simulink model "Simulacion_dinamica_en_DT_export"  (R2023b)
settings: Solver=VariableStepAuto  StartTime=0.0  StopTime=2.5  MaxStep=6e-5  RelTol=1e-3
undefined symbols (not defined in the file): alpha_cu, b_eq, C_ts, id0, J_eq, k_l, L_d, L_ls, L_q, lambda_m, magnitude, P_p, r, R_sREF, R_ts_amb, T_amb, T_sREF
libraries: SignalEditorBlockLib x2, dspsigops x1
settings Model: Creator=tomas  LastModifiedBy=tomas

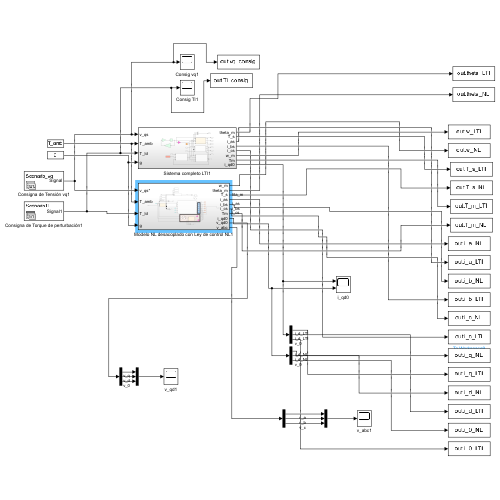
[thumbnail: Simulink's stored preview of the top-level diagram]
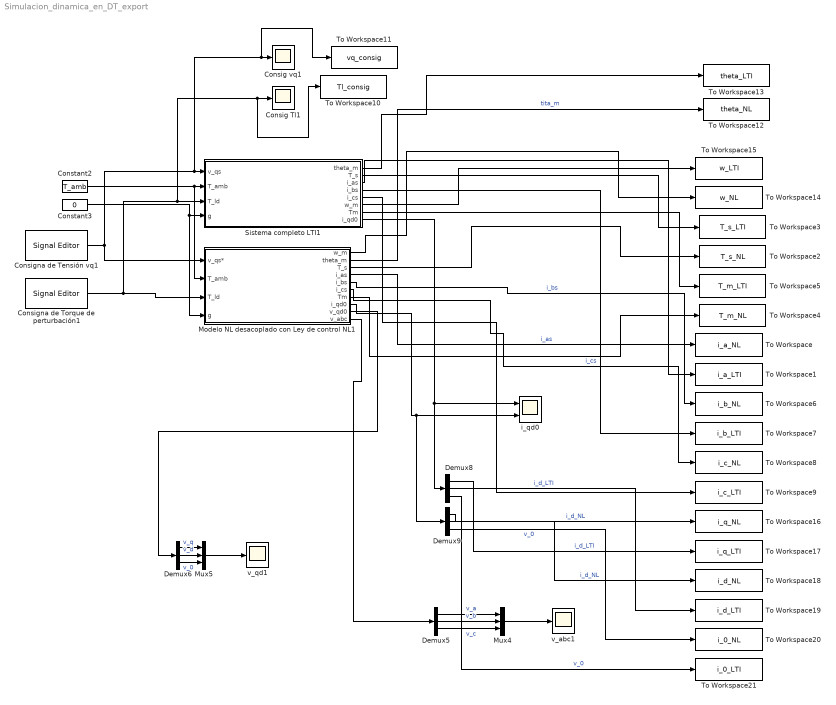
== system Simulacion_dinamica_en_DT_export ==
  Consig Tl1 : Scope
  Consig vq1 : Scope
  Consigna de Tensión vq1 : SignalEditorBlockLib/Signal Editor  FileName=D:\Facu\Final AyME\Final-AyME\Simulink_LA\Simulacion\Señales\senial_vq.mat  ActiveScenario=Scenario_vq  ActiveSignal=Signal  IsBus=off  OutputBusObjectStr=Bus: BusObject  SampleTime=0  Interpolate=off  ZeroCross=off  OutputAfterFinalValue=Setting to zero  Unit=inherit  PreserveSignalName=on  ApplySigPropsToAllScenarios=on  ApplySigPropsToAllSignals=off
  Consigna de Torque de perturbación1 : SignalEditorBlockLib/Signal Editor  FileName=D:\Facu\Final AyME\Final-AyME\Simulink_LA\Simulacion\Señales\Signal_Tl.mat  ActiveScenario=ScenarioTl  ActiveSignal=Signal1  IsBus=off  OutputBusObjectStr=Bus: BusObject  SampleTime=0  Interpolate=off  ZeroCross=off  OutputAfterFinalValue=Setting to zero  Unit=inherit  PreserveSignalName=on  ApplySigPropsToAllScenarios=on  ApplySigPropsToAllSignals=off
  Constant2 : Constant  Value=T_amb
  Constant3 : Constant  Value=0
  Demux{5..6,8..9} (4 alike) : Demux  Outputs=3
  Modelo NL desacoplado con Ley de control NL1 : Subsystem
  Mux4 : Mux  Inputs=3
  Mux5 : Mux  Inputs=3
  Sistema completo LTI1 : Subsystem
  To Workspace : ToWorkspace  VariableName=i_a_NL  SaveFormat=Structure With Time  SampleTime=-1
  To Workspace1 : ToWorkspace  VariableName=i_a_LTI  SaveFormat=Structure With Time  SampleTime=-1
  To Workspace10 : ToWorkspace  VariableName=Tl_consig  SaveFormat=Structure With Time  SampleTime=-1
  To Workspace11 : ToWorkspace  VariableName=vq_consig  SaveFormat=Structure With Time  SampleTime=-1
  To Workspace12 : ToWorkspace  VariableName=theta_NL  SaveFormat=Structure With Time  SampleTime=-1
  To Workspace13 : ToWorkspace  VariableName=theta_LTI  SaveFormat=Structure With Time  SampleTime=-1
  To Workspace14 : ToWorkspace  VariableName=w_NL  SaveFormat=Structure With Time  SampleTime=-1
  To Workspace15 : ToWorkspace  VariableName=w_LTI  SaveFormat=Structure With Time  SampleTime=-1
  To Workspace16 : ToWorkspace  VariableName=i_q_NL  SaveFormat=Structure With Time  SampleTime=-1
  To Workspace17 : ToWorkspace  VariableName=i_q_LTI  SaveFormat=Structure With Time  SampleTime=-1
  To Workspace18 : ToWorkspace  VariableName=i_d_NL  SaveFormat=Structure With Time  SampleTime=-1
  To Workspace19 : ToWorkspace  VariableName=i_d_LTI  SaveFormat=Structure With Time  SampleTime=-1
  To Workspace2 : ToWorkspace  VariableName=T_s_NL  SaveFormat=Structure With Time  SampleTime=-1
  To Workspace20 : ToWorkspace  VariableName=i_0_NL  SaveFormat=Structure With Time  SampleTime=-1
  To Workspace21 : ToWorkspace  VariableName=i_0_LTI  SaveFormat=Structure With Time  SampleTime=-1
  To Workspace3 : ToWorkspace  VariableName=T_s_LTI  SaveFormat=Structure With Time  SampleTime=-1
  To Workspace4 : ToWorkspace  VariableName=T_m_NL  SaveFormat=Structure With Time  SampleTime=-1
  To Workspace5 : ToWorkspace  VariableName=T_m_LTI  SaveFormat=Structure With Time  SampleTime=-1
  To Workspace6 : ToWorkspace  VariableName=i_b_NL  SaveFormat=Structure With Time  SampleTime=-1
  To Workspace7 : ToWorkspace  VariableName=i_b_LTI  SaveFormat=Structure With Time  SampleTime=-1
  To Workspace8 : ToWorkspace  VariableName=i_c_NL  SaveFormat=Structure With Time  SampleTime=-1
  To Workspace9 : ToWorkspace  VariableName=i_c_LTI  SaveFormat=Structure With Time  SampleTime=-1
  i_qd0 : Scope  NumInputPorts=2
  v_abc1 : Scope
  v_qd1 : Scope
  wires:
  Mux4/1 -> v_abc1/1
  Demux5/1 -> Mux4/1  "v_a"
  Sistema completo LTI1/6(w_m) -> To Workspace15/1
  Sistema completo LTI1/4(i_bs) -> To Workspace7/1
  Modelo NL desacoplado con Ley de control NL1/9(v_qd0) -> Demux6/1
  Constant2/1 -> Modelo NL desacoplado con Ley de control NL1/2(T_amb), Sistema completo LTI1/2(T_amb)
  Modelo NL desacoplado con Ley de control NL1/10(v_abc) -> Demux5/1
  Mux5/1 -> v_qd1/1
  Demux6/3 -> Mux5/3  "v_0"
  Demux6/1 -> Mux5/1  "v_q"
  Demux5/2 -> Mux4/2  "v_b"
  Modelo NL desacoplado con Ley de control NL1/7(Tm) -> To Workspace4/1
  Demux5/3 -> Mux4/3  "v_c"
  Modelo NL desacoplado con Ley de control NL1/6(i_cs) -> To Workspace8/1  "i_cs"
  Modelo NL desacoplado con Ley de control NL1/5(i_bs) -> To Workspace6/1  "i_bs"
  Sistema completo LTI1/7(Tm) -> To Workspace5/1
  Modelo NL desacoplado con Ley de control NL1/4(i_as) -> To Workspace/1  "i_as"
  Demux6/2 -> Mux5/2  "v_d"
  Modelo NL desacoplado con Ley de control NL1/1(w_m) -> To Workspace14/1
  Constant3/1 -> Modelo NL desacoplado con Ley de control NL1/4(g), Sistema completo LTI1/4(g)
  Modelo NL desacoplado con Ley de control NL1/2(theta_m) -> To Workspace12/1  "tita_m"
  Sistema completo LTI1/5(i_cs) -> To Workspace9/1
  Modelo NL desacoplado con Ley de control NL1/8(i_qd0) -> i_qd0/2, Demux9/1
  Sistema completo LTI1/8(i_qd0) -> Demux8/1, i_qd0/1
  Sistema completo LTI1/2(T_s) -> To Workspace3/1
  Modelo NL desacoplado con Ley de control NL1/3(T_s) -> To Workspace2/1
  Sistema completo LTI1/1(theta_m) -> To Workspace13/1
  Sistema completo LTI1/3(i_as) -> To Workspace1/1
  Consigna de Tensión vq1/1 -> To Workspace11/1, Consig vq1/1, Sistema completo LTI1/1(v_qs), Modelo NL desacoplado con Ley de control NL1/1(v_qs*)
  Consigna de Torque de perturbación1/1 -> Modelo NL desacoplado con Ley de control NL1/3(T_ld), To Workspace10/1, Consig Tl1/1, Sistema completo LTI1/3(T_ld)
  Demux8/1 -> To Workspace17/1  "i_d_LTI"
  Demux8/2 -> To Workspace19/1  "i_d_LTI"
  Demux8/3 -> To Workspace21/1  "v_0"
  Demux9/1 -> To Workspace16/1  "i_d_NL"
  Demux9/2 -> To Workspace18/1  "i_d_NL"
  Demux9/3 -> To Workspace20/1  "v_0"

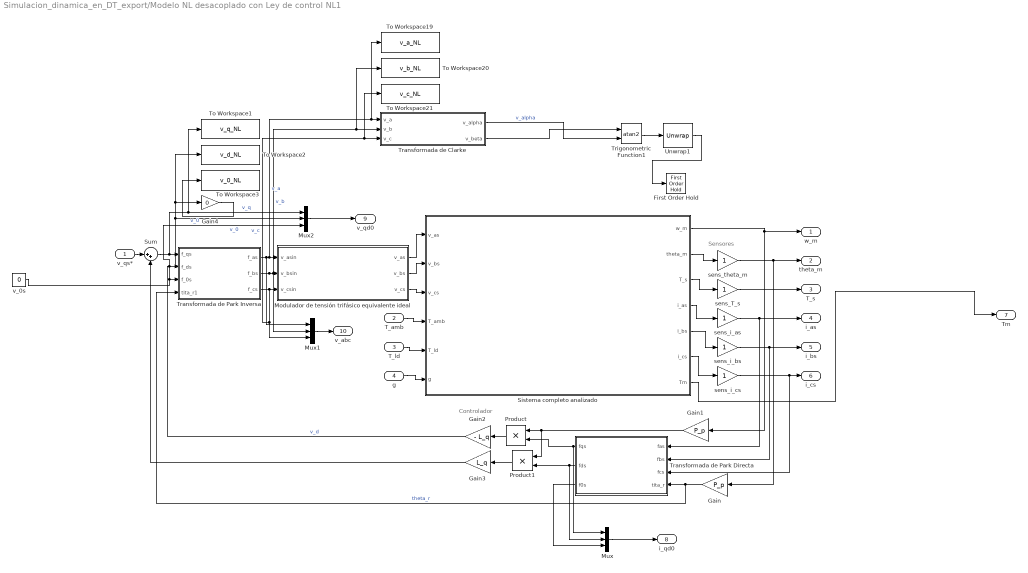
== system Simulacion_dinamica_en_DT_export/Modelo NL desacoplado con Ley de control NL1 ==
  note: Sensores
  note: Controlador
  v_qs* : Inport
  T_amb : Inport  Port=2
  T_ld : Inport  Port=3
  g : Inport  Port=4
  First Order Hold : FirstOrderHold  ErrorTolerance=inf  AllowContinuousInput=on
  Gain : Gain  Gain=P_p
  Gain1 : Gain  Gain=P_p
  Gain2 : Gain  Gain=- L_q
  Gain3 : Gain  Gain=L_q
  Gain4 : Gain  Gain=0
  Modulador de tensión trifásico equivalente ideal : MATLAB Function  TreatAsAtomicUnit=on
  Mux : Mux  Inputs=3
  Mux1 : Mux  Inputs=3
  Mux2 : Mux  Inputs=3
  Product : Product
  Product1 : Product
  "Sistema completo analizado " : Subsystem
  Sum : Sum  Inputs=|++
  To Workspace1 : ToWorkspace  VariableName=v_q_NL  SaveFormat=Structure With Time  SampleTime=-1
  To Workspace19 : ToWorkspace  VariableName=v_a_NL  SaveFormat=Structure With Time  SampleTime=-1
  To Workspace2 : ToWorkspace  VariableName=v_d_NL  SaveFormat=Structure With Time  SampleTime=-1
  To Workspace20 : ToWorkspace  VariableName=v_b_NL  SaveFormat=Structure With Time  SampleTime=-1
  To Workspace21 : ToWorkspace  VariableName=v_c_NL  SaveFormat=Structure With Time  SampleTime=-1
  To Workspace3 : ToWorkspace  VariableName=v_0_NL  SaveFormat=Structure With Time  SampleTime=-1
  Transformada de Clarke : MATLAB Function  TreatAsAtomicUnit=on
  Transformada de Park Directa : Subsystem
  Transformada de Park Inversa : Subsystem
  Trigonometric Function1 : Trigonometry  Operator=atan2
  Unwrap1 : dspsigops/Unwrap  tol=1.2*pi  InputProcessing=Columns as channels (frame based)  running=off
  sens_T_s : Gain
  sens_i_as : Gain
  sens_i_bs : Gain
  sens_i_cs : Gain
  sens_theta_m : Gain
  v_0s : Constant  Value=0
  w_m : Outport
  theta_m : Outport  Port=2
  T_s : Outport  Port=3
  i_as : Outport  Port=4
  i_bs : Outport  Port=5
  i_cs : Outport  Port=6
  Tm : Outport  Port=7
  i_qd0 : Outport  Port=8
  v_qd0 : Outport  Port=9
  v_abc : Outport  Port=10
  wires:
  "Sistema completo analizado "/5(i_bs) -> sens_i_bs/1
  Gain1/1 -> Product1/1, Product/1
  Transformada de Park Directa/3(f0s) -> Mux/3
  T_amb/1 -> "Sistema completo analizado "/4(T_amb)
  "Sistema completo analizado "/3(T_s) -> sens_T_s/1
  g/1 -> "Sistema completo analizado "/6(g)
  Modulador de tensión trifásico equivalente ideal/2(v_bs) -> "Sistema completo analizado "/2(v_bs)
  sens_T_s/1 -> T_s/1
  Transformada de Park Directa/1(fqs) -> Mux/1, Product/2
  Modulador de tensión trifásico equivalente ideal/1(v_as) -> "Sistema completo analizado "/1(v_as)
  sens_i_as/1 -> Transformada de Park Directa/1(fas), i_as/1
  "Sistema completo analizado "/6(i_cs) -> sens_i_cs/1
  "Sistema completo analizado "/4(i_as) -> sens_i_as/1
  Transformada de Park Inversa/3(f_cs) -> Mux1/3, Transformada de Clarke/3(v_c), To Workspace21/1, Modulador de tensión trifásico equivalente ideal/3(v_csin)  "v_c"
  Transformada de Park Inversa/1(f_as) -> Mux1/1, To Workspace19/1, Transformada de Clarke/1(v_a), Modulador de tensión trifásico equivalente ideal/1(v_asin)  "v_a"
  Transformada de Park Inversa/2(f_bs) -> Transformada de Clarke/2(v_b), To Workspace20/1, Mux1/2, Modulador de tensión trifásico equivalente ideal/2(v_bsin)  "v_b"
  v_qs*/1 -> Sum/1
  Product1/1 -> Gain3/1
  "Sistema completo analizado "/2(theta_m) -> sens_theta_m/1
  Transformada de Park Directa/2(fds) -> Mux/2, Product1/2
  sens_theta_m/1 -> Gain/1, theta_m/1
  sens_i_bs/1 -> Transformada de Park Directa/2(fbs), i_bs/1
  v_0s/1 -> Mux2/3, Transformada de Park Inversa/3(f_0s)  "v_0"
  Gain/1 -> Transformada de Park Inversa/4(tita_r1), Transformada de Park Directa/4(tita_r)  "theta_r"
  Gain2/1 -> To Workspace2/1, Gain4/1, Mux2/2, Transformada de Park Inversa/2(f_ds)  "v_d"
  Product/1 -> Gain2/1
  Modulador de tensión trifásico equivalente ideal/3(v_cs) -> "Sistema completo analizado "/3(v_cs)
  Sum/1 -> To Workspace1/1, Mux2/1, Transformada de Park Inversa/1(f_qs)  "v_q"
  sens_i_cs/1 -> Transformada de Park Directa/3(fcs), i_cs/1
  T_ld/1 -> "Sistema completo analizado "/5(T_ld)
  Gain3/1 -> Sum/2
  "Sistema completo analizado "/1(w_m) -> Gain1/1, w_m/1
  "Sistema completo analizado "/7(Tm) -> Tm/1
  Mux/1 -> i_qd0/1
  Mux1/1 -> v_abc/1
  Mux2/1 -> v_qd0/1
  Unwrap1/1 -> First Order Hold/1
  Transformada de Clarke/1(v_alpha) -> Trigonometric Function1/2  "v_alpha"
  Trigonometric Function1/1 -> Unwrap1/1
  Transformada de Clarke/2(v_beta) -> Trigonometric Function1/1
  Gain4/1 -> To Workspace3/1  "v_0"

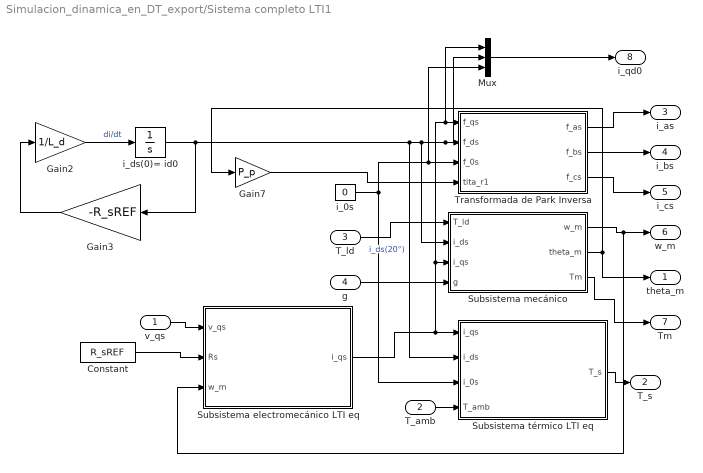
== system Simulacion_dinamica_en_DT_export/Sistema completo LTI1 ==
  v_qs : Inport
  T_amb : Inport  Port=2
  T_ld : Inport  Port=3
  g : Inport  Port=4
  Constant : Constant  Value=R_sREF
  Gain2 : Gain  Gain=1/L_d
  Gain3 : Gain  Gain=-R_sREF
  Gain7 : Gain  Gain=P_p
  Mux : Mux  Inputs=3
  Subsistema electromecánico LTI eq : Subsystem
  Subsistema mecánico : Subsystem
  Subsistema térmico LTI eq : Subsystem
  Transformada de Park Inversa : Subsystem
  i_0s : Constant  Value=0
  i_ds(0)= id0 : Integrator  InitialCondition=id0
  theta_m : Outport
  T_s : Outport  Port=2
  i_as : Outport  Port=3
  i_bs : Outport  Port=4
  i_cs : Outport  Port=5
  w_m : Outport  Port=6
  Tm : Outport  Port=7
  i_qd0 : Outport  Port=8
  wires:
  Subsistema mecánico/2(theta_m) -> theta_m/1, Gain7/1
  v_qs/1 -> Subsistema electromecánico LTI eq/1(v_qs)
  Transformada de Park Inversa/1(f_as) -> i_as/1
  T_ld/1 -> Subsistema mecánico/1(T_ld)
  Transformada de Park Inversa/2(f_bs) -> i_bs/1
  Subsistema térmico LTI eq/1(T_s) -> T_s/1
  Transformada de Park Inversa/3(f_cs) -> i_cs/1
  Subsistema mecánico/1(w_m) -> Subsistema electromecánico LTI eq/3(w_m), w_m/1
  T_amb/1 -> Subsistema térmico LTI eq/4(T_amb)
  i_0s/1 -> Subsistema térmico LTI eq/3(i_0s), Transformada de Park Inversa/3(f_0s), Mux/3
  Constant/1 -> Subsistema electromecánico LTI eq/2(Rs)
  Subsistema electromecánico LTI eq/1(i_qs) -> Subsistema mecánico/3(i_qs), Mux/1, Transformada de Park Inversa/1(f_qs), Subsistema térmico LTI eq/1(i_qs)
  Gain7/1 -> Transformada de Park Inversa/4(tita_r1)
  i_ds(0)= id0/1 -> Subsistema mecánico/2(i_ds), Mux/2, Transformada de Park Inversa/2(f_ds), Subsistema térmico LTI eq/2(i_ds), Gain3/1  "i_ds(20°)"
  Gain2/1 -> i_ds(0)= id0/1  "di/dt"
  g/1 -> Subsistema mecánico/4(g)
  Subsistema mecánico/3(Tm) -> Tm/1
  Mux/1 -> i_qd0/1
  Gain3/1 -> Gain2/1

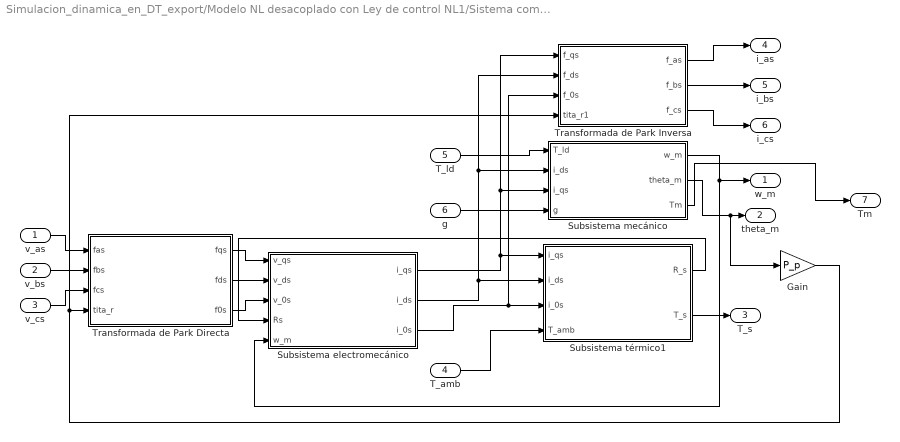
== system Simulacion_dinamica_en_DT_export/Modelo NL desacoplado con Ley de control NL1/Sistema completo analizado  ==
  v_as : Inport
  v_bs : Inport  Port=2
  v_cs : Inport  Port=3
  T_amb : Inport  Port=4
  T_ld : Inport  Port=5
  g : Inport  Port=6
  Gain : Gain  Gain=P_p
  Subsistema electromecánico : Subsystem
  Subsistema mecánico : Subsystem
  Subsistema térmico1 : Subsystem
  Transformada de Park Directa : Subsystem
  Transformada de Park Inversa : Subsystem
  w_m : Outport
  theta_m : Outport  Port=2
  T_s : Outport  Port=3
  i_as : Outport  Port=4
  i_bs : Outport  Port=5
  i_cs : Outport  Port=6
  Tm : Outport  Port=7
  wires:
  Transformada de Park Inversa/3(f_cs) -> i_cs/1
  Subsistema mecánico/1(w_m) -> w_m/1, Subsistema electromecánico/5(w_m)
  Subsistema electromecánico/3(i_0s) -> Subsistema térmico1/3(i_0s), Transformada de Park Inversa/3(f_0s)
  Transformada de Park Directa/1(fqs) -> Subsistema electromecánico/1(v_qs)
  Subsistema térmico1/2(T_s) -> T_s/1
  Transformada de Park Directa/3(f0s) -> Subsistema electromecánico/3(v_0s)
  Subsistema electromecánico/2(i_ds) -> Subsistema térmico1/2(i_ds), Transformada de Park Inversa/2(f_ds), Subsistema mecánico/2(i_ds)
  Gain/1 -> Transformada de Park Inversa/4(tita_r1), Transformada de Park Directa/4(tita_r)
  T_ld/1 -> Subsistema mecánico/1(T_ld)
  Transformada de Park Directa/2(fds) -> Subsistema electromecánico/2(v_ds)
  Transformada de Park Inversa/2(f_bs) -> i_bs/1
  v_bs/1 -> Transformada de Park Directa/2(fbs)
  T_amb/1 -> Subsistema térmico1/4(T_amb)
  Transformada de Park Inversa/1(f_as) -> i_as/1
  v_as/1 -> Transformada de Park Directa/1(fas)
  Subsistema mecánico/2(theta_m) -> Gain/1, theta_m/1
  v_cs/1 -> Transformada de Park Directa/3(fcs)
  Subsistema electromecánico/1(i_qs) -> Transformada de Park Inversa/1(f_qs), Subsistema mecánico/3(i_qs), Subsistema térmico1/1(i_qs)
  Subsistema térmico1/1(R_s) -> Subsistema electromecánico/4(Rs)
  g/1 -> Subsistema mecánico/4(g)
  Subsistema mecánico/3(Tm) -> Tm/1

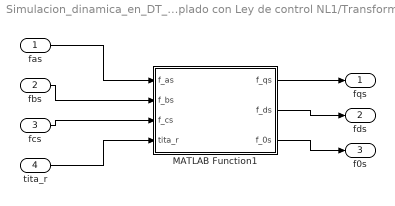
== system Simulacion_dinamica_en_DT_export/Modelo NL desacoplado con Ley de control NL1/Transformada de Park Directa ==
  fas : Inport
  fbs : Inport  Port=2
  fcs : Inport  Port=3
  tita_r : Inport  Port=4
  MATLAB Function1 : MATLAB Function  TreatAsAtomicUnit=on
  fqs : Outport
  fds : Outport  Port=2
  f0s : Outport  Port=3
  wires:
  fas/1 -> MATLAB Function1/1(f_as)
  MATLAB Function1/3(f_0s) -> f0s/1
  MATLAB Function1/2(f_ds) -> fds/1
  fbs/1 -> MATLAB Function1/2(f_bs)
  fcs/1 -> MATLAB Function1/3(f_cs)
  tita_r/1 -> MATLAB Function1/4(tita_r)
  MATLAB Function1/1(f_qs) -> fqs/1

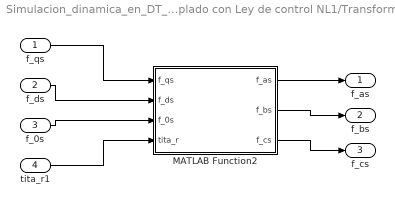
== system Simulacion_dinamica_en_DT_export/Modelo NL desacoplado con Ley de control NL1/Transformada de Park Inversa ==
  f_qs : Inport
  f_ds : Inport  Port=2
  f_0s : Inport  Port=3
  tita_r1 : Inport  Port=4
  MATLAB Function2 : MATLAB Function  TreatAsAtomicUnit=on
  f_as : Outport
  f_bs : Outport  Port=2
  f_cs : Outport  Port=3
  wires:
  tita_r1/1 -> MATLAB Function2/4(tita_r)
  MATLAB Function2/2(f_bs) -> f_bs/1
  MATLAB Function2/1(f_as) -> f_as/1
  f_ds/1 -> MATLAB Function2/2(f_ds)
  MATLAB Function2/3(f_cs) -> f_cs/1
  f_0s/1 -> MATLAB Function2/3(f_0s)
  f_qs/1 -> MATLAB Function2/1(f_qs)

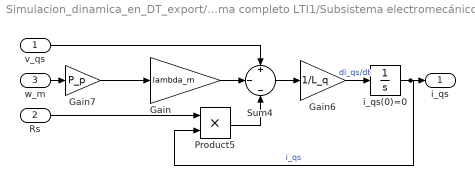
== system Simulacion_dinamica_en_DT_export/Sistema completo LTI1/Subsistema electromecánico LTI eq ==
  v_qs : Inport
  Rs : Inport  Port=2
  w_m : Inport  Port=3
  Gain : Gain  Gain=lambda_m
  Gain6 : Gain  Gain=1/L_q
  Gain7 : Gain  Gain=P_p
  Product5 : Product
  Sum4 : Sum  Inputs=+|-|-
  i_qs(0)=0 : Integrator
  i_qs : Outport
  wires:
  i_qs(0)=0/1 -> Product5/2, i_qs/1  "i_qs"
  v_qs/1 -> Sum4/1
  Gain6/1 -> i_qs(0)=0/1  "di_qs/dt"
  Sum4/1 -> Gain6/1
  Rs/1 -> Product5/1
  w_m/1 -> Gain7/1
  Gain7/1 -> Gain/1
  Product5/1 -> Sum4/3
  Gain/1 -> Sum4/2

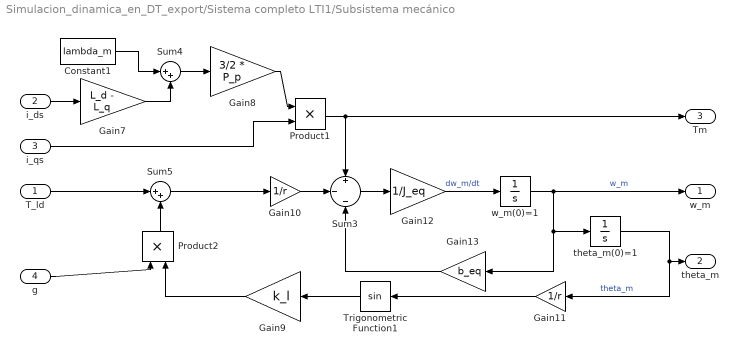
== system Simulacion_dinamica_en_DT_export/Sistema completo LTI1/Subsistema mecánico ==
  T_ld : Inport
  i_ds : Inport  Port=2
  i_qs : Inport  Port=3
  g : Inport  Port=4
  Constant1 : Constant  Value=lambda_m
  Gain10 : Gain  Gain=1/r
  Gain11 : Gain  Gain=1/r
  Gain12 : Gain  Gain=1/J_eq
  Gain13 : Gain  Gain=b_eq
  Gain7 : Gain  Gain=L_d - L_q
  Gain8 : Gain  Gain=3/2 * P_p
  Gain9 : Gain  Gain=k_l
  Product1 : Product
  Product2 : Product
  Sum3 : Sum  Inputs=+|-|-
  Sum4 : Sum  Inputs=|++
  Sum5 : Sum  Inputs=|++
  Trigonometric Function1 : Trigonometry
  theta_m(0)=1 : Integrator
  w_m(0)=1 : Integrator
  w_m : Outport
  theta_m : Outport  Port=2
  Tm : Outport  Port=3
  wires:
  w_m(0)=1/1 -> w_m/1, theta_m(0)=1/1, Gain13/1  "w_m"
  Gain9/1 -> Product2/2
  Gain11/1 -> Trigonometric Function1/1
  i_ds/1 -> Gain7/1
  Constant1/1 -> Sum4/1
  Gain13/1 -> Sum3/3
  Gain10/1 -> Sum3/2
  T_ld/1 -> Sum5/1
  g/1 -> Product2/1
  Trigonometric Function1/1 -> Gain9/1
  theta_m(0)=1/1 -> Gain11/1, theta_m/1  "theta_m"
  Sum5/1 -> Gain10/1
  Product2/1 -> Sum5/2
  Gain8/1 -> Product1/1
  i_qs/1 -> Product1/2
  Sum3/1 -> Gain12/1
  Gain12/1 -> w_m(0)=1/1  "dw_m/dt"
  Sum4/1 -> Gain8/1
  Gain7/1 -> Sum4/2
  Product1/1 -> Sum3/1, Tm/1

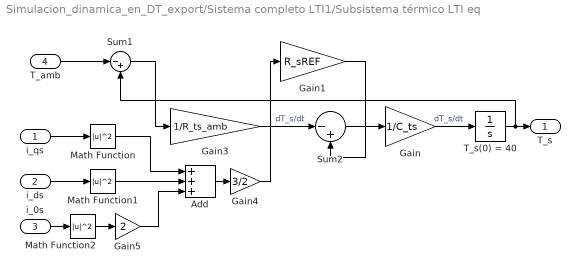
== system Simulacion_dinamica_en_DT_export/Sistema completo LTI1/Subsistema térmico LTI eq ==
  i_qs : Inport
  i_ds : Inport  Port=2
  i_0s : Inport  Port=3
  T_amb : Inport  Port=4
  Add : Sum  Inputs=+++
  Gain : Gain  Gain=1/C_ts
  Gain1 : Gain  Gain=R_sREF
  Gain3 : Gain  Gain=1/R_ts_amb
  Gain4 : Gain  Gain=3/2
  Gain5 : Gain  Gain=2
  Math Function : Math  Operator=magnitude^2
  Math Function1 : Math  Operator=magnitude^2
  Math Function2 : Math  Operator=magnitude^2
  Sum1 : Sum  Inputs=|-+
  Sum2 : Sum  Inputs=|-+
  T_s(0) = 40 : Integrator  InitialCondition=40
  T_s : Outport
  wires:
  Math Function2/1 -> Gain5/1
  Math Function/1 -> Add/1
  T_amb/1 -> Sum1/1
  Sum2/1 -> Gain/1
  Sum1/1 -> Gain3/1
  Gain1/1 -> Sum2/2
  i_ds/1 -> Math Function1/1
  Gain/1 -> T_s(0) = 40/1  "dT_s/dt"
  Gain4/1 -> Gain1/1
  T_s(0) = 40/1 -> Sum1/2, T_s/1
  Math Function1/1 -> Add/2
  i_0s/1 -> Math Function2/1
  Add/1 -> Gain4/1
  Gain5/1 -> Add/3
  i_qs/1 -> Math Function/1
  Gain3/1 -> Sum2/1  "dT_s/dt"

== system Simulacion_dinamica_en_DT_export/Sistema completo LTI1/Transformada de Park Inversa ==
  f_qs : Inport
  f_ds : Inport  Port=2
  f_0s : Inport  Port=3
  tita_r1 : Inport  Port=4
  MATLAB Function2 : MATLAB Function  TreatAsAtomicUnit=on
  f_as : Outport
  f_bs : Outport  Port=2
  f_cs : Outport  Port=3
  wires:
  tita_r1/1 -> MATLAB Function2/4(tita_r)
  MATLAB Function2/2(f_bs) -> f_bs/1
  MATLAB Function2/1(f_as) -> f_as/1
  f_ds/1 -> MATLAB Function2/2(f_ds)
  MATLAB Function2/3(f_cs) -> f_cs/1
  f_0s/1 -> MATLAB Function2/3(f_0s)
  f_qs/1 -> MATLAB Function2/1(f_qs)

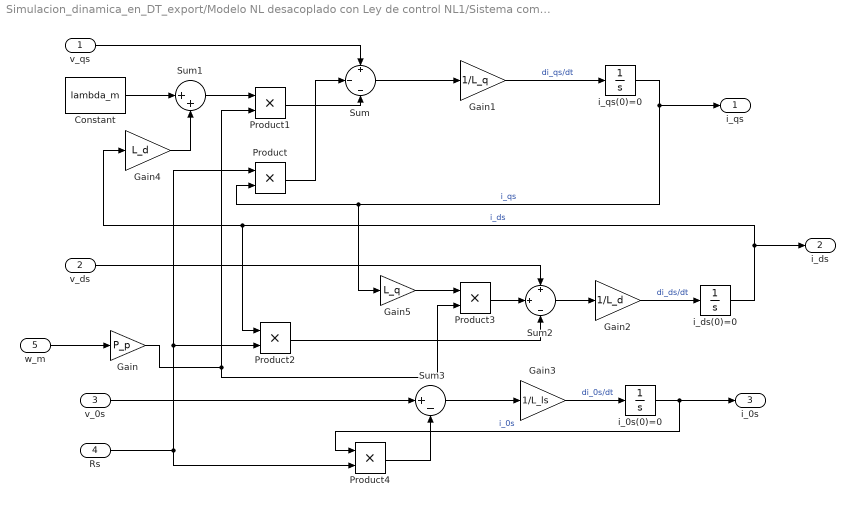
== system Simulacion_dinamica_en_DT_export/Modelo NL desacoplado con Ley de control NL1/Sistema completo analizado /Subsistema electromecánico ==
  v_qs : Inport
  v_ds : Inport  Port=2
  v_0s : Inport  Port=3
  Rs : Inport  Port=4
  w_m : Inport  Port=5
  Constant : Constant  Value=lambda_m
  Gain : Gain  Gain=P_p
  Gain1 : Gain  Gain=1/L_q
  Gain2 : Gain  Gain=1/L_d
  Gain3 : Gain  Gain=1/L_ls
  Gain4 : Gain  Gain=L_d
  Gain5 : Gain  Gain=L_q
  Product{,1..4} (5 alike) : Product
  Sum : Sum  Inputs=+|-|-
  Sum1 : Sum  Inputs=|++
  Sum2 : Sum  Inputs=+|+|-
  Sum3 : Sum  Inputs=|+-
  i_0s(0)=0 : Integrator
  i_ds(0)=0 : Integrator
  i_qs(0)=0 : Integrator
  i_qs : Outport
  i_ds : Outport  Port=2
  i_0s : Outport  Port=3
  wires:
  Gain1/1 -> i_qs(0)=0/1  "di_qs/dt"
  Rs/1 -> Product2/2, Product/1, Product4/2
  i_qs(0)=0/1 -> Gain5/1, Product/2, i_qs/1  "i_qs"
  Sum2/1 -> Gain2/1
  Product1/1 -> Sum/3
  Product4/1 -> Sum3/2
  v_0s/1 -> Sum3/1
  Product3/1 -> Sum2/2
  Gain3/1 -> i_0s(0)=0/1  "di_0s/dt"
  Gain/1 -> Product3/2, Product1/2
  v_qs/1 -> Sum/1
  Sum1/1 -> Product1/1
  Gain5/1 -> Product3/1
  Sum3/1 -> Gain3/1
  i_0s(0)=0/1 -> Product4/1, i_0s/1  "i_0s"
  Product2/1 -> Sum2/3
  Gain2/1 -> i_ds(0)=0/1  "di_ds/dt"
  Constant/1 -> Sum1/1
  Gain4/1 -> Sum1/2
  Sum/1 -> Gain1/1
  Product/1 -> Sum/2
  w_m/1 -> Gain/1
  i_ds(0)=0/1 -> Product2/1, Gain4/1, i_ds/1  "i_ds"
  v_ds/1 -> Sum2/1

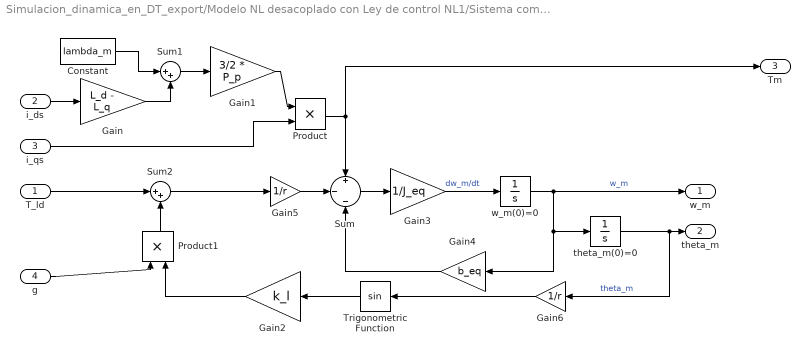
== system Simulacion_dinamica_en_DT_export/Modelo NL desacoplado con Ley de control NL1/Sistema completo analizado /Subsistema mecánico ==
  T_ld : Inport
  i_ds : Inport  Port=2
  i_qs : Inport  Port=3
  g : Inport  Port=4
  Constant : Constant  Value=lambda_m
  Gain : Gain  Gain=L_d - L_q
  Gain1 : Gain  Gain=3/2 * P_p
  Gain2 : Gain  Gain=k_l
  Gain3 : Gain  Gain=1/J_eq
  Gain4 : Gain  Gain=b_eq
  Gain5 : Gain  Gain=1/r
  Gain6 : Gain  Gain=1/r
  Product : Product
  Product1 : Product
  Sum : Sum  Inputs=+|-|-
  Sum1 : Sum  Inputs=|++
  Sum2 : Sum  Inputs=|++
  Trigonometric Function : Trigonometry
  theta_m(0)=0 : Integrator
  w_m(0)=0 : Integrator
  w_m : Outport
  theta_m : Outport  Port=2
  Tm : Outport  Port=3
  wires:
  w_m(0)=0/1 -> w_m/1, theta_m(0)=0/1, Gain4/1  "w_m"
  Sum/1 -> Gain3/1
  Gain3/1 -> w_m(0)=0/1  "dw_m/dt"
  i_ds/1 -> Gain/1
  Constant/1 -> Sum1/1
  Gain/1 -> Sum1/2
  Sum1/1 -> Gain1/1
  Gain1/1 -> Product/1
  i_qs/1 -> Product/2
  Gain4/1 -> Sum/3
  Gain5/1 -> Sum/2
  Trigonometric Function/1 -> Gain2/1
  Gain2/1 -> Product1/2
  theta_m(0)=0/1 -> Gain6/1, theta_m/1  "theta_m"
  T_ld/1 -> Sum2/1
  Sum2/1 -> Gain5/1
  Gain6/1 -> Trigonometric Function/1
  g/1 -> Product1/1
  Product1/1 -> Sum2/2
  Product/1 -> Sum/1, Tm/1

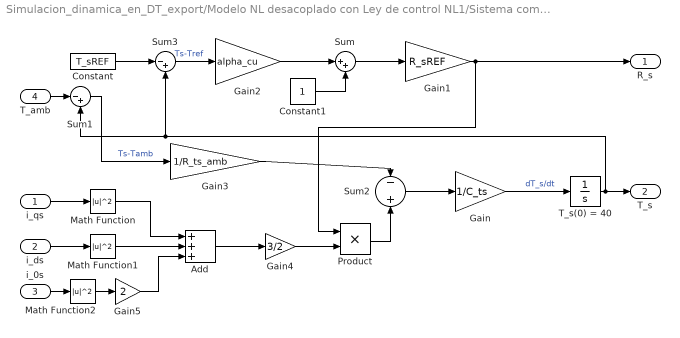
== system Simulacion_dinamica_en_DT_export/Modelo NL desacoplado con Ley de control NL1/Sistema completo analizado /Subsistema térmico1 ==
  i_qs : Inport
  i_ds : Inport  Port=2
  i_0s : Inport  Port=3
  T_amb : Inport  Port=4
  Add : Sum  Inputs=+++
  Constant : Constant  Value=T_sREF
  Constant1 : Constant
  Gain : Gain  Gain=1/C_ts
  Gain1 : Gain  Gain=R_sREF
  Gain2 : Gain  Gain=alpha_cu
  Gain3 : Gain  Gain=1/R_ts_amb
  Gain4 : Gain  Gain=3/2
  Gain5 : Gain  Gain=2
  Math Function : Math  Operator=magnitude^2
  Math Function1 : Math  Operator=magnitude^2
  Math Function2 : Math  Operator=magnitude^2
  Product : Product
  Sum : Sum  Inputs=|++
  Sum1 : Sum  Inputs=|-+
  Sum2 : Sum  Inputs=-|+
  Sum3 : Sum  Inputs=|-+
  T_s(0) = 40 : Integrator  InitialCondition=40
  R_s : Outport
  T_s : Outport  Port=2
  wires:
  Math Function2/1 -> Gain5/1
  Math Function/1 -> Add/1
  T_amb/1 -> Sum1/1
  Sum2/1 -> Gain/1
  Sum/1 -> Gain1/1
  Gain2/1 -> Sum/1
  Gain1/1 -> Product/1, R_s/1
  i_ds/1 -> Math Function1/1
  Gain/1 -> T_s(0) = 40/1  "dT_s/dt"
  Constant1/1 -> Sum/2
  Gain4/1 -> Product/2
  T_s(0) = 40/1 -> T_s/1, Sum3/2, Sum1/2
  Math Function1/1 -> Add/2
  i_0s/1 -> Math Function2/1
  Sum1/1 -> Gain3/1  "Ts-Tamb"
  Add/1 -> Gain4/1
  Gain5/1 -> Add/3
  i_qs/1 -> Math Function/1
  Gain3/1 -> Sum2/1
  Product/1 -> Sum2/2
  Constant/1 -> Sum3/1
  Sum3/1 -> Gain2/1  "Ts-Tref"

== system Simulacion_dinamica_en_DT_export/Modelo NL desacoplado con Ley de control NL1/Sistema completo analizado /Transformada de Park Directa ==
  fas : Inport
  fbs : Inport  Port=2
  fcs : Inport  Port=3
  tita_r : Inport  Port=4
  MATLAB Function1 : MATLAB Function  TreatAsAtomicUnit=on
  fqs : Outport
  fds : Outport  Port=2
  f0s : Outport  Port=3
  wires:
  fas/1 -> MATLAB Function1/1(f_as)
  MATLAB Function1/3(f_0s) -> f0s/1
  MATLAB Function1/2(f_ds) -> fds/1
  fbs/1 -> MATLAB Function1/2(f_bs)
  fcs/1 -> MATLAB Function1/3(f_cs)
  tita_r/1 -> MATLAB Function1/4(tita_r)
  MATLAB Function1/1(f_qs) -> fqs/1

== system Simulacion_dinamica_en_DT_export/Modelo NL desacoplado con Ley de control NL1/Sistema completo analizado /Transformada de Park Inversa ==
  f_qs : Inport
  f_ds : Inport  Port=2
  f_0s : Inport  Port=3
  tita_r1 : Inport  Port=4
  MATLAB Function2 : MATLAB Function  TreatAsAtomicUnit=on
  f_as : Outport
  f_bs : Outport  Port=2
  f_cs : Outport  Port=3
  wires:
  tita_r1/1 -> MATLAB Function2/4(tita_r)
  MATLAB Function2/2(f_bs) -> f_bs/1
  MATLAB Function2/1(f_as) -> f_as/1
  f_ds/1 -> MATLAB Function2/2(f_ds)
  MATLAB Function2/3(f_cs) -> f_cs/1
  f_0s/1 -> MATLAB Function2/3(f_0s)
  f_qs/1 -> MATLAB Function2/1(f_qs)

== matlab function Simulacion_dinamica_en_DT_export/Modelo NL desacoplado con Ley de control NL1/Modulador de tensión trifásico equivalente ideal ==
  data: v_asin input; v_as output; v_bsin input; v_csin input; v_bs output; v_cs output
function [v_as,v_bs,v_cs] = ModuladorIdeal(v_asin,v_bsin, v_csin)
v_as=v_asin;
v_bs=v_bsin;
v_cs=v_csin;

== matlab function Simulacion_dinamica_en_DT_export/Modelo NL desacoplado con Ley de control NL1/Sistema completo analizado /Transformada de Park Directa/MATLAB Function1 ==
  data: f_as input; f_qs output; f_bs input; f_cs input; tita_r input; f_ds output; f_0s output
function [f_qs, f_ds, f_0s] = parkDir(f_as,f_bs,f_cs,tita_r)

answer = 2/3 * [cos(tita_r), cos(tita_r - 2*pi/3), cos(tita_r + 2*pi/3);
         sin(tita_r), sin(tita_r - 2*pi/3), sin(tita_r + 2*pi/3);
         1/2, 1/2, 1/2] * [f_as;f_bs;f_cs];

f_qs = answer(1);
f_ds = answer(2);
f_0s = answer(3);

== matlab function Simulacion_dinamica_en_DT_export/Modelo NL desacoplado con Ley de control NL1/Sistema completo analizado /Transformada de Park Inversa/MATLAB Function2 ==
  data: f_qs input; f_as output; f_ds input; f_0s input; tita_r input; f_bs output; f_cs output
function [f_as, f_bs, f_cs] = parkInv(f_qs,f_ds,f_0s,tita_r)

answer = [cos(tita_r), sin(tita_r), 1;
         cos(tita_r - 2*pi/3), sin(tita_r - 2*pi/3), 1;
         cos(tita_r + 2*pi/3), sin(tita_r + 2*pi/3), 1] * [f_qs;f_ds;f_0s]; 

f_as = answer(1);
f_bs = answer(2);
f_cs = answer(3);

== matlab function Simulacion_dinamica_en_DT_export/Modelo NL desacoplado con Ley de control NL1/Transformada de Clarke ==
  data: v_a input; v_alpha output; v_b input; v_c input; v_beta output
function [v_alpha,v_beta] = Clarke_Transform(v_a,v_b, v_c)
v_alpha=(2/3)*(v_a - 0.5*(v_a+v_b));
v_beta=(sqrt(3)/3)*(v_b-v_c);

== matlab function Simulacion_dinamica_en_DT_export/Modelo NL desacoplado con Ley de control NL1/Transformada de Park Directa/MATLAB Function1 ==
  data: f_as input; f_qs output; f_bs input; f_cs input; tita_r input; f_ds output; f_0s output
function [f_qs, f_ds, f_0s] = parkDir(f_as,f_bs,f_cs,tita_r)

answer = 2/3 * [cos(tita_r), cos(tita_r - 2*pi/3), cos(tita_r + 2*pi/3);
         sin(tita_r), sin(tita_r - 2*pi/3), sin(tita_r + 2*pi/3);
         1/2, 1/2, 1/2] * [f_as;f_bs;f_cs];

f_qs = answer(1);
f_ds = answer(2);
f_0s = answer(3);

== matlab function Simulacion_dinamica_en_DT_export/Modelo NL desacoplado con Ley de control NL1/Transformada de Park Inversa/MATLAB Function2 ==
  data: f_qs input; f_as output; f_ds input; f_0s input; tita_r input; f_bs output; f_cs output
function [f_as, f_bs, f_cs] = parkInv(f_qs,f_ds,f_0s,tita_r)

answer = [cos(tita_r), sin(tita_r), 1;
         cos(tita_r - 2*pi/3), sin(tita_r - 2*pi/3), 1;
         cos(tita_r + 2*pi/3), sin(tita_r + 2*pi/3), 1] * [f_qs;f_ds;f_0s]; 

f_as = answer(1);
f_bs = answer(2);
f_cs = answer(3);

== matlab function Simulacion_dinamica_en_DT_export/Sistema completo LTI1/Transformada de Park Inversa/MATLAB Function2 ==
  data: f_qs input; f_as output; f_ds input; f_0s input; tita_r input; f_bs output; f_cs output
function [f_as, f_bs, f_cs] = parkInv(f_qs,f_ds,f_0s,tita_r)

answer = [cos(tita_r), sin(tita_r), 1;
         cos(tita_r - 2*pi/3), sin(tita_r - 2*pi/3), 1;
         cos(tita_r + 2*pi/3), sin(tita_r + 2*pi/3), 1] * [f_qs;f_ds;f_0s]; 

f_as = answer(1);
f_bs = answer(2);
f_cs = answer(3);
